simulink model "Unbatch1_Model"  (R2024b)
settings: Solver=VariableStepAuto  StartTime=0.0  StopTime=10.0  RelTol=1e-3
libraries: NSA_DEVS_LOGISTICS x6, NSA_DEVS_SINKS x3, NSA_DEVS_SOURCES x1
settings Model: Creator=david  LastModifiedBy=peter
settings RTWCC: GPUComputeCapability=3.5

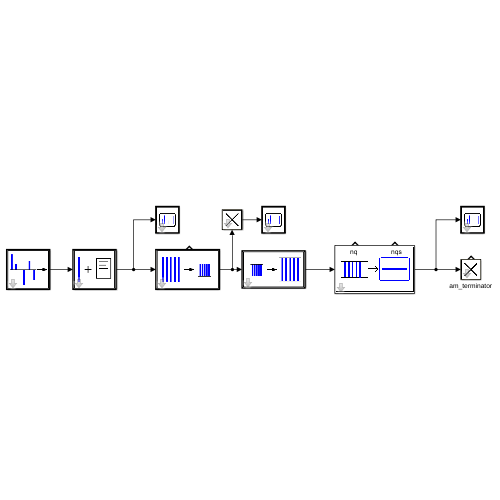
[thumbnail: Simulink's stored preview of the top-level diagram]
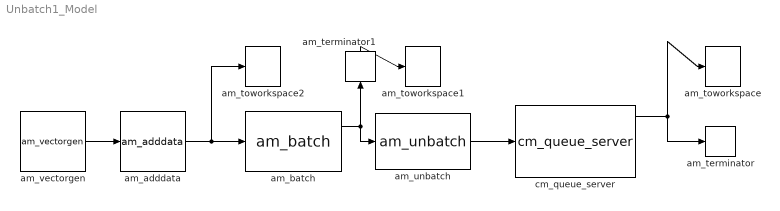
== system Unbatch1_Model ==
  am_adddata : NSA_DEVS_LOGISTICS/am_adddata  fields=[]  values=[]  numeric=[]  infield="\"value\""  tau=[0,1]  debug=0
      settings: SourceProductName=Logistics
  am_batch : NSA_DEVS_LOGISTICS/am_batch  N=2  tau=[0,1]  debug=0
      settings: SourceProductName=Logistics
  am_terminator : NSA_DEVS_LOGISTICS/am_terminator  tau=[0,1]  debug=0
      settings: SourceProductName=Logistics
  am_terminator1 : NSA_DEVS_LOGISTICS/am_terminator  tau=[0,1]  debug=0
      settings: SourceProductName=Logistics
  am_toworkspace : NSA_DEVS_SINKS/am_toworkspace  varname="\"out\""  t0=0  format="\"vector\""  tau=[0,0.5]  debug=0
      settings: SourceProductName=Sinks
  am_toworkspace1 : NSA_DEVS_SINKS/am_toworkspace  varname="\"batch\""  t0=0  format="\"vector\""  tau=[0,0.5]  debug=0
      settings: SourceProductName=Sinks
  am_toworkspace2 : NSA_DEVS_SINKS/am_toworkspace  varname="\"in\""  t0=0  format="\"vector\""  tau=[0,0.5]  debug=0
      settings: SourceProductName=Sinks
  am_unbatch : NSA_DEVS_LOGISTICS/am_unbatch  tD=[0,2]  tau=[0,1]  debug=0
      settings: SourceProductName=Logistics
  am_vectorgen : NSA_DEVS_SOURCES/am_vectorgen  tvec=1:6  yvec=[1 3 1 2 2 2]  tau=[0,1]  debug=0
      settings: SourceProductName=Sources
  cm_queue_server : NSA_DEVS_LOGISTICS/cm_queue_server  ts=0.1  tau=[0,1]  debug=0
      settings: SourceProductName=Logistics
  wires:
  am_batch/1 -> am_terminator1/1, am_unbatch/1
  am_vectorgen/1 -> am_adddata/1
  am_adddata/1 -> am_toworkspace2/1, am_batch/1
  am_terminator1/1 -> am_toworkspace1/1
  am_unbatch/1 -> cm_queue_server/1
  cm_queue_server/1 -> am_toworkspace/1, am_terminator/1
